simulink model "hextodec_file"  (R2018b)
settings: Solver=VariableStepAuto  StartTime=0.0  StopTime=10.0  RelTol=1e-3
settings Model: Creator=Saliou  LastModifiedBy=Saliou

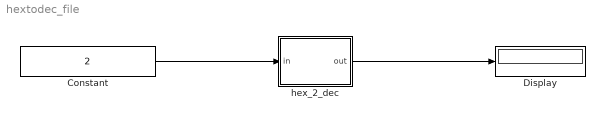
== system hextodec_file ==
  Constant : Constant  Value=2
  Display : Display
  hex_2_dec : MATLAB Function  TreatAsAtomicUnit=on
  wires:
  Constant/1 -> hex_2_dec/1(in)
  hex_2_dec/1(out) -> Display/1

== matlab function hextodec_file/hex_2_dec ==
  data: in input; out output
function out = hextodec(in)

out = hex2dec ('in');
